simulink model "complementary_filter"  (R2019a)
settings: Solver=VariableStepAuto  StartTime=0.0  StopTime=26  RelTol=1e-3
values from neighbouring files (symbols this model uses):
  acc_bias = [mean(Rx_ax(1:40)); mean(Rx_ay(1:40)); mean(Rx_az(1:40))]    [VLP_method_2d_h.m]    (also in VLP_method_comparison.m; VLP_method_comparison_stats.m)
settings Model: Creator=LENOVO  LastModifiedBy=LENOVO

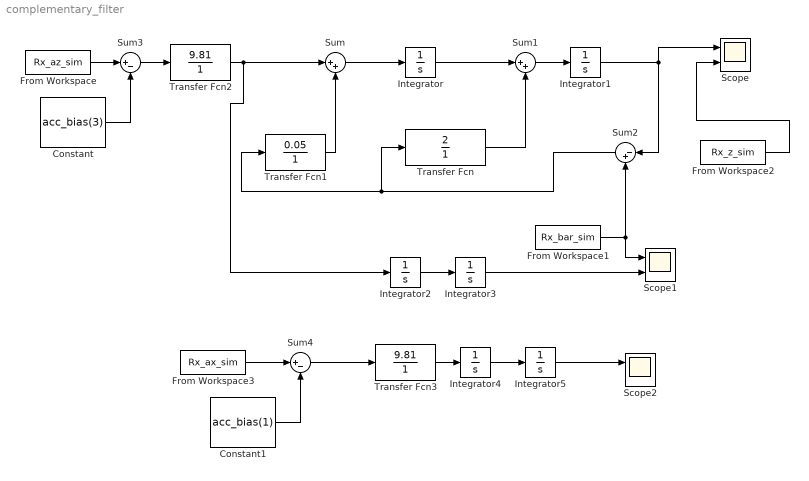
== system complementary_filter ==
  Constant : Constant  Value=acc_bias(3)
  Constant1 : Constant  Value=acc_bias(1)
  From Workspace : FromWorkspace  VariableName=Rx_az_sim  SampleTime=0
  From Workspace1 : FromWorkspace  VariableName=Rx_bar_sim  SampleTime=0
  From Workspace2 : FromWorkspace  VariableName=Rx_z_sim  SampleTime=0
  From Workspace3 : FromWorkspace  VariableName=Rx_ax_sim  SampleTime=0
  Integrator{,1..5} (6 alike) : Integrator
  Scope : Scope  NumInputPorts=2
  Scope1 : Scope  NumInputPorts=2
  Scope2 : Scope  NumInputPorts=2
  Sum : Sum  Inputs=|++
  Sum1 : Sum  Inputs=|++
  Sum2 : Sum  Inputs=|-+
  Sum3 : Sum  Inputs=|+-
  Sum4 : Sum  Inputs=|+-
  Transfer Fcn : TransferFcn  Numerator=[2]  Denominator=[1]
  Transfer Fcn1 : TransferFcn  Numerator=[0.05]  Denominator=[1]
  Transfer Fcn2 : TransferFcn  Numerator=[9.81]  Denominator=[1]
  Transfer Fcn3 : TransferFcn  Numerator=[9.81]  Denominator=[1]
  wires:
  Sum/1 -> Integrator/1
  Integrator/1 -> Sum1/1
  Sum1/1 -> Integrator1/1
  Integrator1/1 -> Scope/1, Sum2/1
  From Workspace1/1 -> Scope1/1, Sum2/2
  Sum2/1 -> Transfer Fcn1/1, Transfer Fcn/1
  Transfer Fcn/1 -> Sum1/2
  Transfer Fcn1/1 -> Sum/2
  From Workspace2/1 -> Scope/2
  From Workspace/1 -> Sum3/1
  Transfer Fcn2/1 -> Integrator2/1, Sum/1
  Sum3/1 -> Transfer Fcn2/1
  Constant/1 -> Sum3/2
  Integrator3/1 -> Scope1/2
  Integrator2/1 -> Integrator3/1
  Integrator5/1 -> Scope2/1
  Integrator4/1 -> Integrator5/1
  Sum4/1 -> Transfer Fcn3/1
  From Workspace3/1 -> Sum4/1
  Constant1/1 -> Sum4/2
  Transfer Fcn3/1 -> Integrator4/1
